simulink model "tracking"  (R2016b)
settings: Solver=VariableStepAuto  StartTime=0.0  StopTime=inf  RelTol=1e-3
undefined symbols (not defined in the file or in its folder): gray, Horn, Rec, Schunck, SDTV, strel, videoinput
libraries: visionstatistics x3, visionmorphops x1, visionconversions x1, visiontextngfix x1, imaqlib x1, visionanalysis x1
settings Model: Creator=Anushri-MacBook  LastModifiedBy=Anushri-MacBook

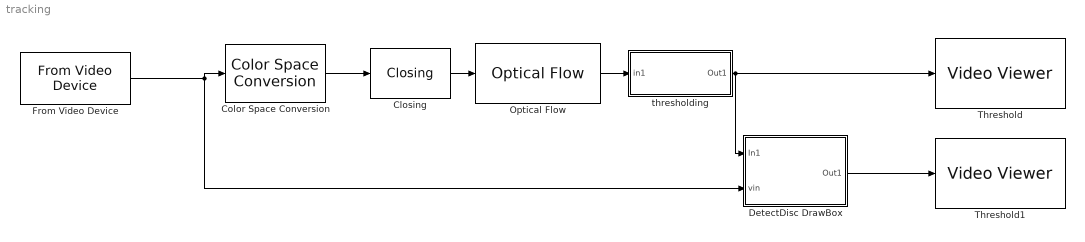
== system tracking ==
  Closing : visionmorphops/Closing  nhoodsrc=Specify via dialog  strel=strel('line',5,45)
  Color Space Conversion : visionconversions/Color Space  Conversion  conversion=Obsolete  conversionActive=R'G'B' to intensity  wp_str=D65  rec=Rec. 601 (SDTV)  sys=1125/60/2:1  imagePorts=One multidimensional signal
  "DetectDisc DrawBox " : Subsystem
  From Video Device : imaqlib/From Video Device  DeviceMenu=macvideo 1 (FaceTime HD Camera)  Device=macvideo 1 (FaceTime HD Camera)  ObjConstructor=videoinput('macvideo', 1)  VideoFormatMenu=YCbCr422_1280x720  VideoFormat=YCbCr422_1280x720  VideoSource=default  ROIPosition=[0 0 720 1280]  EnableHWTrigger=off  TriggerConfiguration=macvideo 1 (FaceTime HD Camera)  SampleTime=1/30  OutputPortsMode=One multidimensional signal  DataType=single  CanDoHWTrigger=no  ReturnedColorSpace=rgb  BlockHandle=1713.0005  ROIWidth=1280  ROIHeight=720  ROIColumn=0  ROIRow=0  EngXMLPath=/Applications/MATLAB_R2016b.app/toolbox/imaq/imaq/private  DevXMLPath=/Users/Anushri-MacBook/Documents/MATLAB/SupportPackages/R2016b/toolbox/imaq/supportpackages/genericvideo/adaptor/maci64  EngLibPath=/Applications/MATLAB_R2016b.app/toolbox/imaq/imaqblks/imaqmex/maci64  ColorSpace=rgb  BayerSensorAlignment=grbg
  Optical Flow : visionanalysis/Optical Flow  method=Horn-Schunck  gradMethod=Difference filter [-1 1]  which2img=Current frame and N-th frame back  N=1  outVelForm=Magnitude-squared  lambda=1  stop_criteria=When maximum number of iterations is reached  maxAllowAbsDiff=eps  maxIter=15  numInports=3  sigmaS=1.5  sigmaW=1  eigTh=0.0039  discardNormalFlow=off  outputCurrentImage=off  prodOutputMode=Binary point scaling  prodOutputWordLength=32  prodOutputFracLength=20  outputMode=Binary point scaling  outputWordLength=32  outputFracLength=20  roundingMode=Nearest  overflowMode=on
  Threshold : VideoViewer  colormapValue=gray(256)  FigPos=[73 649 611 548]  trueSizedOnce=on
  Threshold1 : VideoViewer  colormapValue=gray(256)  FigPos=[707 729 734 604]  trueSizedOnce=on
  thresholding : Subsystem
  wires:
  Optical Flow/1 -> thresholding/1(in1)
  thresholding/1(Out1) -> Threshold/1, "DetectDisc DrawBox "/1(In1)
  "DetectDisc DrawBox "/1(Out1) -> Threshold1/1
  Color Space Conversion/1 -> Closing/1
  Closing/1 -> Optical Flow/1
  From Video Device/1 -> Color Space Conversion/1, "DetectDisc DrawBox "/2(vin)

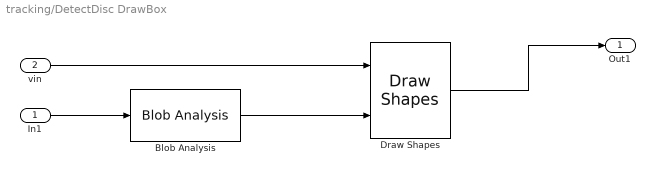
== system tracking/DetectDisc DrawBox  ==
  In1 : Inport
  vin : Inport  Port=2
  Blob Analysis : visionstatistics/Blob Analysis  Tag=vipblks_row_conv  area=off  centroid=off  bBox=on  majorAxis=off  minorAxis=off  angle=off  eccentricity=off  equivDiameterSq=off  extent=off  perimeter=off  maxBlobs=5  warnIfNumBlobsExceeded=on  isCount=off  useMinArea=on  minArea=300  useMaxArea=on  maxArea=700  excludeBorderBlob=on  outDT=double  isOutVarDim=on  isFill=on  fillValues=-1  conn=8  isLabel=off  outputMode=Binary point scaling  outputWordLength=32  outputFracLength=16  firstCoeffMode=Binary point scaling  firstCoeffWordLength=16  firstCoeffFracLength=14  secondCoeffMode=Binary point scaling  secondCoeffWordLength=32  secondCoeffFracLength=16  accumMode=Binary point scaling  accumWordLength=32  accumFracLength=0  prodOutputMode=Binary point scaling  prodOutputWordLength=32  prodOutputFracLength=16  roundingMode=Floor  overflowMode=off
  Draw Shapes : visiontextngfix/Draw Shapes  shape=Rectangles  fill=off  lineWidth=1  fillClrSource=Specify via dialog  display=User-specified value  intensity=200  color=[0 1 0]  opacity=0.6  viewport=Entire image  antialiasing=off  inType=Obsolete  imagePorts=One multidimensional signal  prodOutputMode=Binary point scaling  prodOutputWordLength=32  prodOutputFracLength=14  memoryMode=Specify word length  memoryWordLength=16  memoryFracLength=15  roundingMode=Floor  overflowMode=off
  Out1 : Outport
  wires:
  In1/1 -> Blob Analysis/1
  Blob Analysis/1 -> Draw Shapes/2
  vin/1 -> Draw Shapes/1
  Draw Shapes/1 -> Out1/1

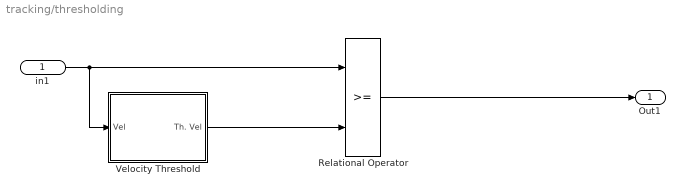
== system tracking/thresholding ==
  in1 : Inport
  Relational Operator : RelationalOperator  OutDataTypeStr=boolean  RndMeth=Nearest
  Velocity Threshold : Subsystem
  Out1 : Outport
  wires:
  in1/1 -> Velocity Threshold/1(Vel), Relational Operator/1
  Relational Operator/1 -> Out1/1
  Velocity Threshold/1(Th. Vel) -> Relational Operator/2

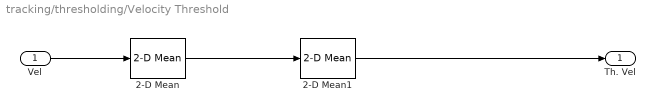
== system tracking/thresholding/Velocity Threshold ==
  Vel : Inport
  2-D Mean : visionstatistics/2-D Mean  run=off  reset_popup=None  directionMode=Entire input  dimension=1  treatSBRowAsCol=on  roiEnable=off  roiType=Rectangles  roiPortion=Entire ROI  roiOutput=Individual statistics for each ROI  roiFlag=off  outputDataTypeStr=Inherit: Same as accumulator  outputLastDataTypeStr=Inherit: Same as accumulator  outputMin=[]  outputMax=[]  accumMode=Binary point scaling  accumWordLength=32  accumFracLength=0  accumDataTypeStr=fixdt([],32,0)  accumLastDataTypeStr=fixdt([],32,0)  roundingMode=Floor  overflowMode=off
  2-D Mean1 : visionstatistics/2-D Mean  run=on  reset_popup=None  directionMode=Entire input  dimension=1  treatSBRowAsCol=on  roiEnable=off  roiType=Rectangles  roiPortion=Entire ROI  roiOutput=Individual statistics for each ROI  roiFlag=off  outputDataTypeStr=Inherit: Same as accumulator  outputLastDataTypeStr=Inherit: Same as accumulator  outputMin=[]  outputMax=[]  accumMode=Binary point scaling  accumWordLength=32  accumFracLength=0  accumDataTypeStr=fixdt([],32,0)  accumLastDataTypeStr=fixdt([],32,0)  roundingMode=Floor  overflowMode=off
  Th. Vel : Outport
  wires:
  2-D Mean/1 -> 2-D Mean1/1
  Vel/1 -> 2-D Mean/1
  2-D Mean1/1 -> Th. Vel/1
